simulink model "eserciziosimulink3_5"  (R2020b)
settings: Solver=FixedStepAuto  StartTime=0.0  StopTime=tfin  FixedStep=1e-1  RelTol=1e-9  AbsTol=1e-9  EnableMultiTasking=on
values from neighbouring files (symbols this model uses):
  Q0 = angle2quat(psi0,theta0,phi0)    [PRELooping_SIM.m]    (also in PRETonneau_SIM.m)
  xe0 = 0    [PRELooping_SIM.m]    (also in PRETonneau_SIM.m)
  ye0 = 0    [PRELooping_SIM.m]    (also in PRETonneau_SIM.m)
  ze0 = 0    [PRELooping_SIM.m]    (also in PRETonneau_SIM.m)
libraries: sharedtransform x2, aerolibconvert2 x1
settings Model: Creator=antoi  LastModifiedBy=isido
settings SolverCC: AutoScaleAbsTol=off  ZeroCrossControl=DisableAll
settings DataIOCC: LimitDataPoints=on  ReturnWorkspaceOutputs=off
settings OptimizationCC: LifeSpan=inf
settings DebuggingCC: AllowSymbolicDim=off  SFUnexpectedBacktrackingDiag=warning  SFNoUnconditionalDefaultTransitionDiag=warning  ArithmeticOperatorsInVariantConditions=warning
settings ModelReferenceCC: PropagateSignalLabelsOutOfModel=off
settings SFSimCC: SimUseLocalCustomCode=off  CustomCodeUndefinedFunction=UseInterfaceOnly
settings RTWCC: RTWUseLocalCustomCode=off
settings CodeAppCC: StateflowObjectComments=on
settings GRTTargetCC: TargetLangStandard=C89/C90 (ANSI)
settings ConfigComp: CovMetricSettings=dw  CovSaveCumulativeToWorkspaceVar=on  CovSaveSingleToWorkspaceVar=on  CovExternalEMLEnable=off

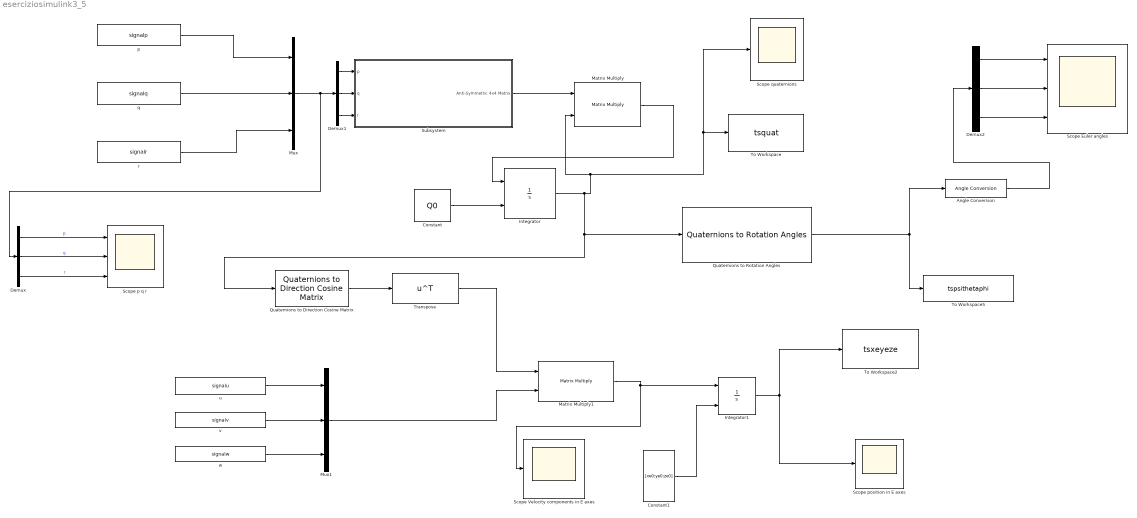
== system eserciziosimulink3_5 ==
  Angle Conversion : aerolibconvert2/Angle Conversion  IU=rad  OU=deg
  Constant : Constant  Value=Q0
  Constant1 : Constant  Value=[xe0;ye0;ze0]  VectorParams1D=off
  Demux : Demux  Outputs=3
  Demux1 : Demux  Outputs=3
  Demux2 : Demux  Outputs=3
  Integrator : Integrator  InitialConditionSource=external  ContinuousStateAttributes='quat'
  Integrator1 : Integrator  InitialConditionSource=external  AbsoluteTolerance=10^-9  ContinuousStateAttributes='PositionE'
  Matrix Multiply : Product  Inputs=**  Multiplication=Matrix(*)
  Matrix Multiply1 : Product  Inputs=**  Multiplication=Matrix(*)
  Mux : Mux  Inputs=3
  Mux1 : Mux  Inputs=3
  Quaternions to Direction Cosine Matrix : sharedtransform/Quaternions to  Direction Cosine Matrix  aMode=aMode
      settings: SourceProductBaseCode=AE,PW,MT,UV,VE,VP
  Quaternions to Rotation Angles : sharedtransform/Quaternions to Rotation Angles  rotationOrder=ZYX  aMode=aMode
      settings: SourceProductBaseCode=AE,PW,MT,UV,VE,VP
  Scope Euler angles : Scope  NumInputPorts=3
  Scope Velocity components in E axes : Scope
  Scope p q r : Scope  NumInputPorts=3
  Scope position in E axes : Scope
  Scope quaternions : Scope
  Subsystem : Subsystem
  To Workspace : ToWorkspace  VariableName=tsquat  SaveFormat=Timeseries  SampleTime=-1
  To Workspace2 : ToWorkspace  VariableName=tsxeyeze  SaveFormat=Timeseries  SampleTime=-1
  To Workspace5 : ToWorkspace  VariableName=tspsithetaphi  SaveFormat=Timeseries  SampleTime=-1
  Transpose : Math  Operator=transpose  SignedPower=on  SaturateOnIntegerOverflow=on
  p : FromWorkspace  VariableName=signalp  OutputAfterFinalValue=Setting to zero
  q : FromWorkspace  VariableName=signalq  OutputAfterFinalValue=Setting to zero
  r : FromWorkspace  VariableName=signalr  OutputAfterFinalValue=Setting to zero
  u : FromWorkspace  VariableName=signalu  OutputAfterFinalValue=Holding final value
  v : FromWorkspace  VariableName=signalv  OutputAfterFinalValue=Holding final value
  w : FromWorkspace  VariableName=signalw  OutputAfterFinalValue=Holding final value
  wires:
  Mux/1 -> Demux1/1, Demux/1
  Demux/1 -> Scope p q r/1  "p"
  Demux/2 -> Scope p q r/2  "q"
  Demux/3 -> Scope p q r/3  "r"
  Demux1/1 -> Subsystem/1(p)
  Demux1/2 -> Subsystem/2(q)
  Demux1/3 -> Subsystem/3(r)
  Subsystem/1(Anti-Symmetric 4x4 Matrix) -> Matrix Multiply/1
  Constant/1 -> Integrator/2
  Matrix Multiply/1 -> Integrator/1
  Integrator/1 -> Quaternions to Direction Cosine Matrix/1, Quaternions to Rotation Angles/1, Scope quaternions/1, To Workspace/1, Matrix Multiply/2
  Quaternions to Direction Cosine Matrix/1 -> Transpose/1
  Transpose/1 -> Matrix Multiply1/1
  Mux1/1 -> Matrix Multiply1/2
  Matrix Multiply1/1 -> Integrator1/1, Scope Velocity components in E axes/1
  Constant1/1 -> Integrator1/2
  Integrator1/1 -> To Workspace2/1, Scope position in E axes/1
  Angle Conversion/1 -> Demux2/1
  Quaternions to Rotation Angles/1 -> To Workspace5/1, Angle Conversion/1
  Demux2/1 -> Scope Euler angles/1
  Demux2/2 -> Scope Euler angles/2
  Demux2/3 -> Scope Euler angles/3
  q/1 -> Mux/2
  r/1 -> Mux/3
  p/1 -> Mux/1
  u/1 -> Mux1/1
  v/1 -> Mux1/2
  w/1 -> Mux1/3

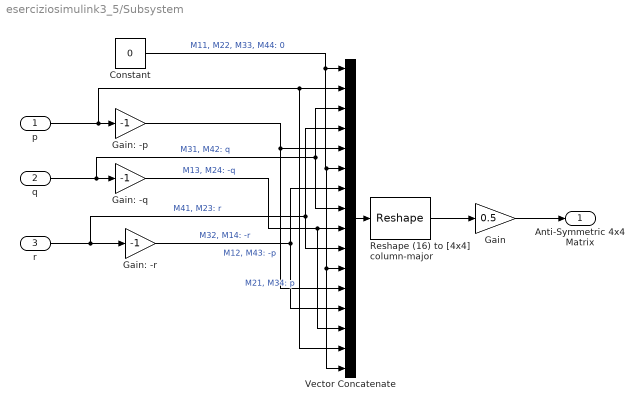
== system eserciziosimulink3_5/Subsystem ==
  p : Inport  PortDimensions=1
  q : Inport  Port=2  PortDimensions=1
  r : Inport  Port=3  PortDimensions=1
  Constant : Constant  Value=0
  Gain : Gain  Gain=0.5
  Gain: -p : Gain  Gain=-1
  Gain: -q : Gain  Gain=-1
  Gain: -r : Gain  Gain=-1
  Reshape (16) to [4x4] column-major : Reshape  OutputDimensionality=Customize  OutputDimensions=[4,4]
  Vector Concatenate : Concatenate  NumInputs=16
  Anti-Symmetric 4x4 Matrix : Outport  PortDimensions=[4 4]
  wires:
  Constant/1 -> Vector Concatenate/16, Vector Concatenate/11, Vector Concatenate/6, Vector Concatenate/1  "M11, M22, M33, M44: 0"
  p/1 -> Vector Concatenate/15, Vector Concatenate/2, Gain: -p/1  "M21, M34: p"
  Gain: -q/1 -> Vector Concatenate/14, Vector Concatenate/9  "M13, M24: -q"
  Gain: -p/1 -> Vector Concatenate/12, Vector Concatenate/5  "M12, M43: -p"
  r/1 -> Vector Concatenate/10, Vector Concatenate/4, Gain: -r/1  "M41, M23: r"
  Gain: -r/1 -> Vector Concatenate/13, Vector Concatenate/7  "M32, M14: -r"
  q/1 -> Vector Concatenate/3, Vector Concatenate/8, Gain: -q/1  "M31, M42: q"
  Vector Concatenate/1 -> Reshape (16) to [4x4] column-major/1
  Reshape (16) to [4x4] column-major/1 -> Gain/1
  Gain/1 -> Anti-Symmetric 4x4 Matrix/1
